simulink model "Ejemplo"  (R2017b)
settings: Solver=ode2  StartTime=0.0  StopTime=20  FixedStep=0.001  RelTol=1e-3
libraries: simulink x2
settings Model: Creator=Marco  LastModifiedBy=Marco
settings SolverCC: AlgebraicLoopSolver=LineSearch

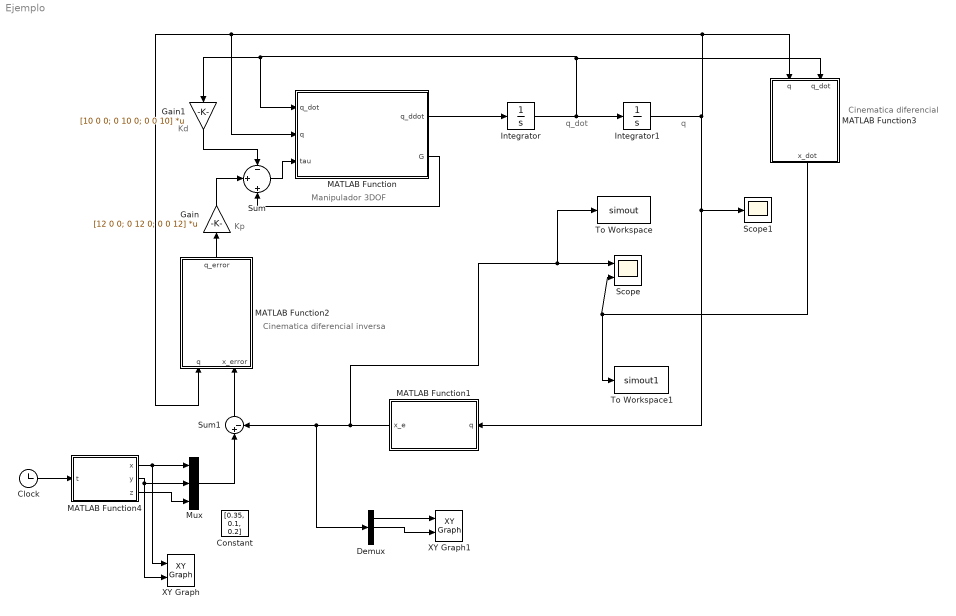
== system Ejemplo ==
  note: Cinematica diferencial
  note: Cinematica diferencial inversa
  note: Kd
  note: Kp
  note: Manipulador 3DOF
  note: q
  note: q_dot
  Clock : Clock
  Constant : Constant  Value=[0.35, 0.1, 0.2]
  Demux : Demux  Outputs=3
  Gain : Gain  Gain=[12 0 0; 0 12 0; 0 0 12]  Multiplication=Matrix(K*u)
  Gain1 : Gain  Gain=[10 0 0; 0 10 0; 0 0 10]  Multiplication=Matrix(K*u)
  Integrator : Integrator  InitialCondition=[0; 0; 0]
  Integrator1 : Integrator  InitialCondition=[0; 1.45; 1]
  MATLAB Function : MATLAB Function  TreatAsAtomicUnit=on
  MATLAB Function1 : MATLAB Function  TreatAsAtomicUnit=on
  MATLAB Function2 : MATLAB Function  TreatAsAtomicUnit=on
  MATLAB Function3 : MATLAB Function  TreatAsAtomicUnit=on
  MATLAB Function4 : MATLAB Function  TreatAsAtomicUnit=on
  Mux : Mux  Inputs=3
  Scope : Scope  NumInputPorts=2
  Scope1 : Scope
  Sum : Sum  Inputs=-|+|+
  Sum1 : Sum  Inputs=|+-
  To Workspace : ToWorkspace  VariableName=simout  SaveFormat=Timeseries  SampleTime=-1
  To Workspace1 : ToWorkspace  VariableName=simout1  SaveFormat=Timeseries  SampleTime=-1
  XY Graph : simulink/Sinks/XY Graph  xmin=-0.3  xmax=0.4  ymin=-0.3  ymax=0.4  st=-1
  XY Graph1 : simulink/Sinks/XY Graph  xmin=-0.3  xmax=0.4  ymin=-0.3  ymax=0.4  st=-1
  wires:
  MATLAB Function/1(q_ddot) -> Integrator/1
  Sum/1 -> MATLAB Function/3(tau)
  Integrator/1 -> MATLAB Function3/2(q_dot), Gain1/1, MATLAB Function/1(q_dot), Integrator1/1
  MATLAB Function/2(G) -> Sum/3
  MATLAB Function1/1(x_e) -> To Workspace/1, Scope/1, Demux/1, Sum1/2
  Sum1/1 -> MATLAB Function2/2(x_error)
  Gain/1 -> Sum/2
  MATLAB Function2/1(q_error) -> Gain/1
  Gain1/1 -> Sum/1
  MATLAB Function3/1(x_dot) -> To Workspace1/1, Scope/2
  Clock/1 -> MATLAB Function4/1(t)
  MATLAB Function4/1(x) -> Mux/1, XY Graph/1
  MATLAB Function4/2(y) -> Mux/2, XY Graph/2
  Integrator1/1 -> Scope1/1, MATLAB Function1/1(q), MATLAB Function3/1(q), MATLAB Function2/1(q), MATLAB Function/2(q)
  MATLAB Function4/3(z) -> Mux/3
  Mux/1 -> Sum1/1
  Demux/1 -> XY Graph1/1
  Demux/2 -> XY Graph1/2

== matlab function Ejemplo/MATLAB Function1 ==
  data: q input; x_e output
function x_e = CinematicaDirecta(q)

l2 = 0.3;
l3 = 0.3;

x_e = [l2*cos(q(2)) + l3*cos(q(2))*cos(q(3));
       l3*sin(q(3));
       q(1) + l2*sin(q(2)) + l3*cos(q(3))*sin(q(2))];
end

== matlab function Ejemplo/MATLAB Function ==
  data: q_dot input; q input; q_ddot output; tau input; G output
function [q_ddot, G]= manipulador(q_dot,q,tau)
%Valores del robot
g = 9.81; %m/s^2
l2 = 0.3; %m
lc2 = 0.15; %m
lc3 = 0.15; %m
m1 = 0.2; %Kg
m2 = 0.2; %Kg
m3 = 0.2; %Kg
I2 = 0.001; %Kg*m^2
I3 = 0.001; %Kg*m^2

%---------------------------Matriz de Inercias----------------------------%
m11 = m1/4 + m2 + m3;
m12 = lc2*m2*cos(q(2)) + m3*cos(q(2))*(l2 + lc3*cos(q(3)));
m13 = lc3*m3*sin(q(2))*sin(q(3));
m21 = lc2*m2*cos(q(2)) + m3*cos(q(2))*(l2 + lc3*cos(q(3)));
m22 = I2 + I3 + (l2^2)*m3 + (lc2^2)*m2 + (lc3^2)*m3*cos(q(3))^2 + 2*l2*lc3*m3*cos(q(3));
m23 = 0;
m31 = -lc3*m3*sin(q(2))*sin(q(3));
m32 = 0; 
m33 = m3*(lc3^2) + I3;

M = [m11 m12 m13;
     m21 m22 m23;
     m31 m32 m33];
%----------------------------Matriz de Coriolis---------------------------%

c11 = 0;
c12 = - q_dot(2)*(lc2*m2*sin(q(2)) + m3*sin(q(2))*(l2 + lc3*cos(q(3)))) - lc3*m3*q_dot(3)*cos(q(2))*sin(q(3));
c13 = -lc3*m3*(q_dot(2)*cos(q(2))*sin(q(3)) + q_dot(3)*cos(q(3))*sin(q(2)));
c21 = 0;
c22 = -(lc3*m3*q_dot(3)*(lc3*sin(2*q(3)) + 2*l2*sin(q(3))))/2;
c23 = -(lc3*m3*q_dot(2)*(lc3*sin(2*q(3)) + 2*l2*sin(q(3))))/2;
c31 = 0;
c32 = (lc3*m3*q_dot(1)*(lc3*sin(2*q(3)) + 2*l2*sin(q(3))))/2;
c33 = 0;

C = [c11 c12 c13;
     c21 c22 c23;
     c31 c32 c33];
%----------------------------Vector de Gravedad---------------------------%
g11 = g*((m1/2)+m2+m3);
g21 = g*(lc3*m3*cos(q(3))+l2*m3+lc2*m2)*cos(q(2));
g31 = -g*lc3*m3*sin(q(2))*sin(q(3));

G = [g11;
     g21;
     g31];
 
q_ddot = M\(tau-C*q_dot-G);

== matlab function Ejemplo/MATLAB Function2 ==
  data: q input; q_error output; x_error input
function q_error = Inv_J(q,x_error)

l2 = 0.3;
l3 = 0.3;

Inv_J = [cos(q(2))/sin(q(2)), sin(q(3))/(cos(q(3))*sin(q(2))), 1;
         -1/(sin(q(2))*(l2 + l3*cos(q(3)))), -(cos(q(2))*sin(q(3)))/(cos(q(3))*sin(q(2))*(l2 + l3*cos(q(3)))), 0;
          0, 1/(l3*cos(q(3))), 0];
      
q_error = Inv_J*x_error;

end

== matlab function Ejemplo/MATLAB Function3 ==
  data: q input; x_dot output; q_dot input
function x_dot = J(q,q_dot)

l2 = 0.3;
l3 = 0.3;

J = [0, -sin(q(2))*(l2 + l3*cos(q(3))), -l3*cos(q(2))*sin(q(3));
     0, 0, l3*cos(q(3));
     1, cos(q(2))*(l2 + l3*cos(q(3))), -l3*sin(q(2))*sin(q(3))];

x_dot = J*q_dot;

== matlab function Ejemplo/MATLAB Function4 ==
  data: x output; t input; y output; z output
function [x, y, z] = trayectoria(t)

x = (0.5+sin(t)^3)*0.25;
y = (0.5+cos(t)^3)*0.25;
z = 0.4;

% if (t<=6)
% x = 0.35;
% y = 0.1;
% z = 0.4;  
% elseif ((t>6)&&(t<=12))
% x = 0;
% y = 0.3;
% z = 0.4;
% elseif ((t>12)&&(t<=18))
% x = -0.35;
% y = 0.1;
% z = 0.4;
% elseif ((t>18)&&(t<=24))
% x = -0.3;
% y = -0.3;
% z = 0.4;
% else
% x = 0.3;
% y = -0.3;
% z = 0.4;
% end

end
